simulink model "ptension"  (Simulink 3.00)
settings: Solver=ode4  SolverMode=SingleTasking  StartTime=0.0  StopTime=2.355  FixedStep=0.001  MaxStep=0.001  RelTol=1e-3  AbsTol=1e-3
values from neighbouring files (symbols this model uses):
  b = 5E-5    (= 5e-05)    [Constants.m]
  J = 1    [Constants.m]
  Ka = 20    [Constants.m]
  Ke = 1.356    [Constants.m]
  Km = 1.36    [Constants.m]
  Kp = 50    [Constants.m]
  Kt = 0.0955    [Constants.m]
  R = 0.37    [Constants.m]
settings Model: SaveTime=off  SaveOutput=off

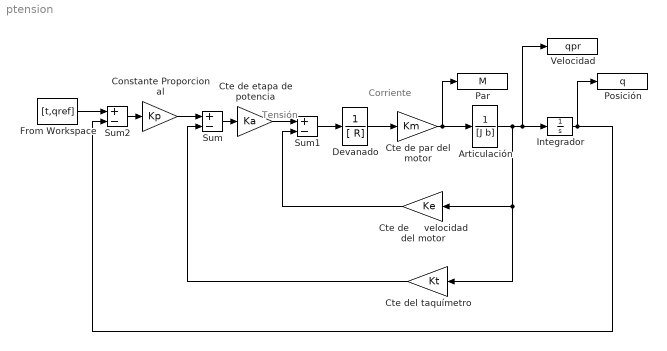
== system ptension ==
  note: Tensión
  note: Corriente
  Articulación : TransferFcn  Numerator=[1]  Denominator=[J b]
  Constante Proporcional : Gain  Gain=Kp  SaturateOnIntegerOverflow=on
  Cte de etapa de potencia : Gain  Gain=Ka  SaturateOnIntegerOverflow=on
  Cte de par del motor : Gain  Gain=Km  SaturateOnIntegerOverflow=on
  Cte de     velocidad del motor : Gain  Orientation=left  Gain=Ke  SaturateOnIntegerOverflow=on
  Cte del taquímetro : Gain  Orientation=left  Gain=Kt  SaturateOnIntegerOverflow=on
  Devanado : TransferFcn  Numerator=[1]  Denominator=[ R]
  From Workspace : FromWorkspace  VariableName=[t,qref]  SampleTime=0.001  HoldFinalValue=off
  Integrador : Integrator  ExternalReset=none  InitialConditionSource=internal  InitialCondition=0  LimitOutput=off  UpperSaturationLimit=inf  LowerSaturationLimit=-inf  ShowSaturationPort=off  ShowStatePort=off  AbsoluteTolerance=auto
  Par : ToWorkspace  VariableName=M  SampleTime=0  SaveFormat=Matrix
      settings: Buffer=2335
  Posición : ToWorkspace  VariableName=q  SampleTime=0  SaveFormat=Matrix
      settings: Buffer=2335
  Sum : Sum  Inputs=+-  SaturateOnIntegerOverflow=on
  Sum1 : Sum  Inputs=+-  SaturateOnIntegerOverflow=on
  Sum2 : Sum  Inputs=+-  SaturateOnIntegerOverflow=on
  Velocidad : ToWorkspace  VariableName=qpr  SampleTime=0  SaveFormat=Matrix
      settings: Buffer=2335
  wires:
  Sum/1 -> Cte de etapa de potencia/1
  Sum1/1 -> Devanado/1
  Devanado/1 -> Cte de par del motor/1
  Cte de etapa de potencia/1 -> Sum1/1
  Cte de     velocidad del motor/1 -> Sum1/2
  Cte del taquímetro/1 -> Sum/2
  Constante Proporcional/1 -> Sum/1
  Sum2/1 -> Constante Proporcional/1
  From Workspace/1 -> Sum2/1
  Articulación/1 -> Cte del taquímetro/1, Cte de     velocidad del motor/1, Integrador/1, Velocidad/1
  Cte de par del motor/1 -> Articulación/1, Par/1
  Integrador/1 -> Sum2/2, Posición/1
